simulink model "baselineisp_ref_imp_v1"  (R2023b)
settings: Solver=VariableStepAuto  StartTime=0.0  StopTime=0  RelTol=1e-3
undefined symbols (not defined in the file): gray, ispdata, ispdatainfo
libraries: visionconversions x1, visionanalysis x1
settings Model: Creator=csl  LastModifiedBy=csl

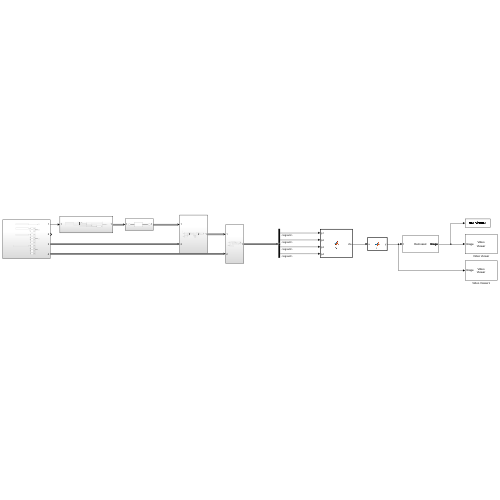
[thumbnail: Simulink's stored preview of the top-level diagram]
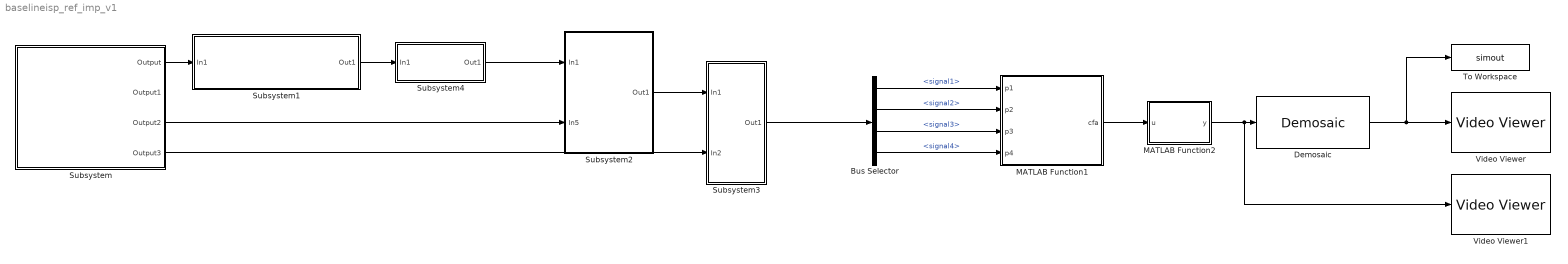
== system baselineisp_ref_imp_v1 ==
  Bus Selector : BusSelector  OutputSignals=signal1,signal2,signal3,signal4
  Demosaic : visionconversions/Demosaic  algorithm=Obsolete  algorithmActive=Bilinear  alignment=BGGR  imagePorts=One multidimensional signal  roundingMode=Floor  overflowMode=on  prodOutputMode=Binary point scaling  prodOutputWordLength=32  prodOutputFracLength=10
  MATLAB Function1 : MATLAB Function  TreatAsAtomicUnit=on
  MATLAB Function2 : MATLAB Function  TreatAsAtomicUnit=on
  Subsystem : Subsystem
  Subsystem1 : Subsystem
  Subsystem2 : Subsystem
  Subsystem3 : Subsystem
  Subsystem4 : Subsystem
  To Workspace : ToWorkspace  VariableName=simout  SaveFormat=Timeseries
  Video Viewer : VideoViewer  colormapValue=gray(256)  FigPos=[1 1078 1093 766]
  Video Viewer1 : VideoViewer  colormapValue=gray(256)  FigPos=[1 1078 1093 766]
  wires:
  Subsystem/3(Output2) -> Subsystem2/2(In5)
  Subsystem2/1(Out1) -> Subsystem3/1(In1)
  Subsystem/4(Output3) -> Subsystem3/2(In2)
  Subsystem3/1(Out1) -> Bus Selector/1
  Bus Selector/1 -> MATLAB Function1/1(p1)  "<signal1>"
  Bus Selector/2 -> MATLAB Function1/2(p2)  "<signal2>"
  Bus Selector/3 -> MATLAB Function1/3(p3)  "<signal3>"
  Bus Selector/4 -> MATLAB Function1/4(p4)  "<signal4>"
  MATLAB Function2/1(y) -> Video Viewer1/1, Demosaic/1
  MATLAB Function1/1(cfa) -> MATLAB Function2/1(u)
  Demosaic/1 -> Video Viewer/1, To Workspace/1
  Subsystem1/1(Out1) -> Subsystem4/1(In1)
  Subsystem/1(Output) -> Subsystem1/1(In1)
  Subsystem4/1(Out1) -> Subsystem2/1(In1)

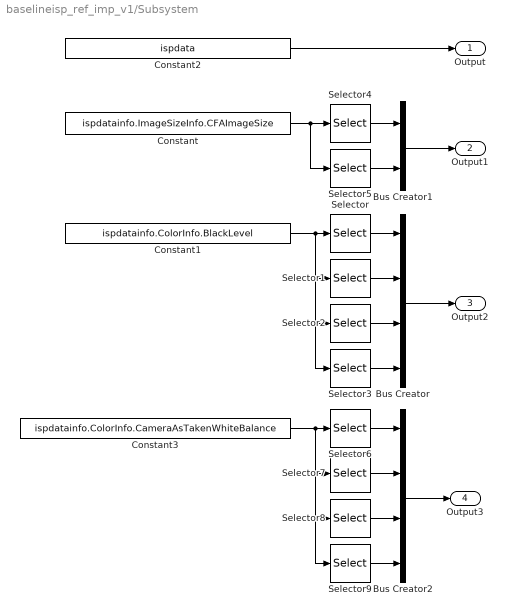
== system baselineisp_ref_imp_v1/Subsystem ==
  Bus Creator : BusCreator  Inputs=4
  Bus Creator1 : BusCreator  Inputs=2
  Bus Creator2 : BusCreator  Inputs=4
  Constant : Constant  Value=ispdatainfo.ImageSizeInfo.CFAImageSize
  Constant1 : Constant  Value=ispdatainfo.ColorInfo.BlackLevel  OutDataTypeStr=uint16
  Constant2 : Constant  Value=ispdata  OutDataTypeStr=uint16
  Constant3 : Constant  Value=ispdatainfo.ColorInfo.CameraAsTakenWhiteBalance  OutDataTypeStr=double
  Selector : Selector  NumberOfDimensions=2  InputPortWidth=3  IndexOptions=Index vector (dialog),Index vector (dialog)  Indices=1,1  OutputSizes=1,1
  Selector1 : Selector  NumberOfDimensions=2  InputPortWidth=3  IndexOptions=Index vector (dialog),Index vector (dialog)  Indices=1,2  OutputSizes=1,1
  Selector2 : Selector  NumberOfDimensions=2  InputPortWidth=3  IndexOptions=Index vector (dialog),Index vector (dialog)  Indices=2,1  OutputSizes=1,1
  Selector3 : Selector  NumberOfDimensions=2  InputPortWidth=3  IndexOptions=Index vector (dialog),Index vector (dialog)  Indices=2,2  OutputSizes=1,1
  Selector4 : Selector  InputPortWidth=2  IndexOptions=Index vector (dialog)  Indices=1  OutputSizes=1
  Selector5 : Selector  InputPortWidth=2  IndexOptions=Index vector (dialog)  Indices=2  OutputSizes=1
  Selector6 : Selector  InputPortWidth=4  IndexOptions=Index vector (dialog)  Indices=1  OutputSizes=1
  Selector7 : Selector  InputPortWidth=4  IndexOptions=Index vector (dialog)  Indices=2  OutputSizes=1
  Selector8 : Selector  InputPortWidth=4  IndexOptions=Index vector (dialog)  Indices=3  OutputSizes=1
  Selector9 : Selector  InputPortWidth=4  IndexOptions=Index vector (dialog)  Indices=4  OutputSizes=1
  Output : Outport
  Output1 : Outport  Port=2
  Output2 : Outport  Port=3
  Output3 : Outport  Port=4
  wires:
  Selector/1 -> Bus Creator/1
  Selector1/1 -> Bus Creator/2
  Selector2/1 -> Bus Creator/3
  Selector3/1 -> Bus Creator/4
  Constant1/1 -> Selector3/1, Selector2/1, Selector1/1, Selector/1
  Selector4/1 -> Bus Creator1/1
  Selector5/1 -> Bus Creator1/2
  Constant/1 -> Selector5/1, Selector4/1
  Bus Creator1/1 -> Output1/1
  Bus Creator/1 -> Output2/1
  Constant2/1 -> Output/1
  Selector6/1 -> Bus Creator2/1
  Selector7/1 -> Bus Creator2/2
  Selector8/1 -> Bus Creator2/3
  Selector9/1 -> Bus Creator2/4
  Constant3/1 -> Selector9/1, Selector8/1, Selector7/1, Selector6/1
  Bus Creator2/1 -> Output3/1

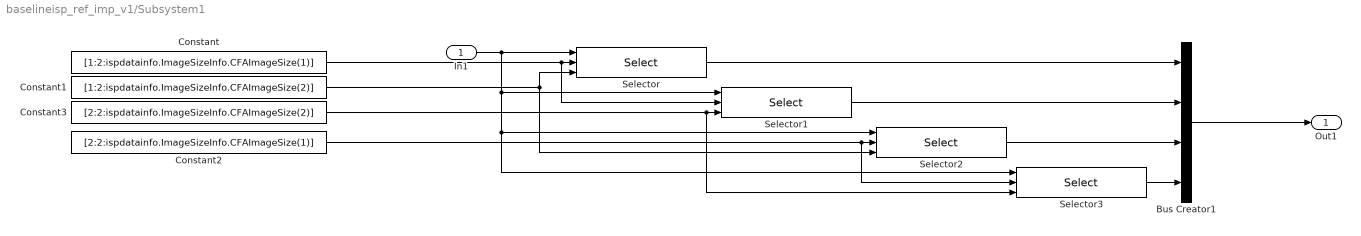
== system baselineisp_ref_imp_v1/Subsystem1 ==
  In1 : Inport
  Bus Creator1 : BusCreator  Inputs=4
  Constant : Constant  Value=[1:2:ispdatainfo.ImageSizeInfo.CFAImageSize(1)]
  Constant1 : Constant  Value=[1:2:ispdatainfo.ImageSizeInfo.CFAImageSize(2)]
  Constant2 : Constant  Value=[2:2:ispdatainfo.ImageSizeInfo.CFAImageSize(1)]
  Constant3 : Constant  Value=[2:2:ispdatainfo.ImageSizeInfo.CFAImageSize(2)]
  Selector{,1..3} (4 alike) : Selector  NumberOfDimensions=2  InputPortWidth=3  IndexOptions=Index vector (port),Index vector (port)  Indices=[1 3],1  OutputSizes=1,1
  Out1 : Outport
  wires:
  Selector1/1 -> Bus Creator1/2
  Selector2/1 -> Bus Creator1/3
  Bus Creator1/1 -> Out1/1
  Selector/1 -> Bus Creator1/1
  Selector3/1 -> Bus Creator1/4
  In1/1 -> Selector/1, Selector2/1, Selector3/1, Selector1/1
  Constant/1 -> Selector1/2, Selector/2
  Constant1/1 -> Selector/3, Selector2/3
  Constant3/1 -> Selector3/3, Selector1/3
  Constant2/1 -> Selector3/2, Selector2/2

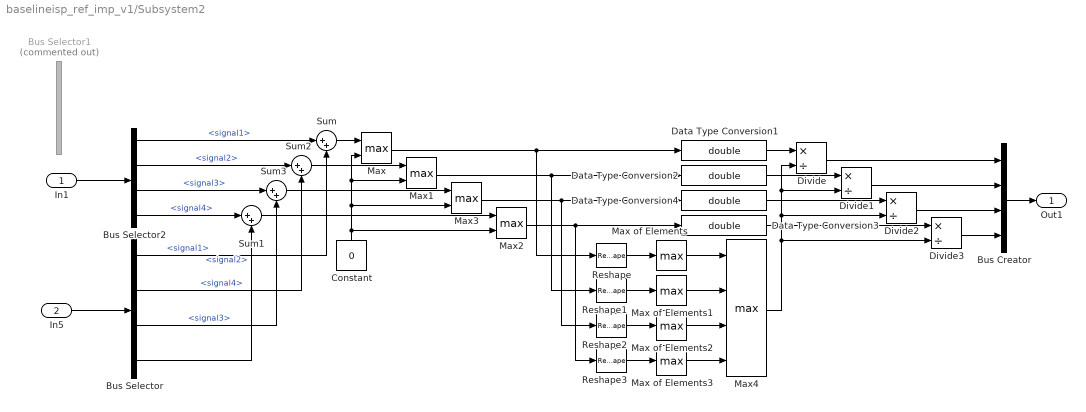
== system baselineisp_ref_imp_v1/Subsystem2 ==
  In1 : Inport
  In5 : Inport  Port=2
  Bus Creator : BusCreator  Inputs=4
  Bus Selector : BusSelector  OutputSignals=signal1,signal4,signal3,signal2
  Bus Selector1 : BusSelector  Commented=on  OutputSignals=p1,p2,p3,p4
  Bus Selector2 : BusSelector  OutputSignals=signal1,signal2,signal3,signal4
  Constant : Constant  Value=0
  Data Type Conversion{1..4} (4 alike) : DataTypeConversion  OutDataTypeStr=double  SaturateOnIntegerOverflow=off  RndMeth=Floor
  Divide{,1..3} (4 alike) : Product  Inputs=*/
  Max{,1..3} (4 alike) : MinMax  Function=max  Inputs=2
  Max of Elements{,1..3} (4 alike) : MinMax  Function=max
  Max4 : MinMax  Function=max  Inputs=4
  Reshape{,1..3} (4 alike) : Reshape
  Sum{,1..3} (4 alike) : Sum  Inputs=|++
  Out1 : Outport
  wires:
  Bus Selector/3 -> Sum3/2  "<signal3>"
  In5/1 -> Bus Selector/1
  Bus Selector/1 -> Sum/2  "<signal1>"
  Bus Selector2/2 -> Sum2/1  "<signal2>"
  Bus Selector/2 -> Sum2/2  "<signal4>"
  Bus Selector2/3 -> Sum3/1  "<signal3>"
  Bus Selector2/4 -> Sum1/1  "<signal4>"
  Bus Selector/4 -> Sum1/2  "<signal2>"
  Bus Selector2/1 -> Sum/1  "<signal1>"
  Bus Creator/1 -> Out1/1
  In1/1 -> Bus Selector2/1
  Sum/1 -> Max/1
  Sum2/1 -> Max1/1
  Sum3/1 -> Max3/1
  Sum1/1 -> Max2/1
  Max/1 -> Reshape/1, Data Type Conversion1/1
  Max1/1 -> Data Type Conversion2/1, Reshape1/1
  Max3/1 -> Data Type Conversion4/1, Reshape2/1
  Max2/1 -> Data Type Conversion3/1, Reshape3/1
  Constant/1 -> Max3/2, Max1/2, Max/2, Max2/2
  Reshape/1 -> Max of Elements/1
  Reshape1/1 -> Max of Elements1/1
  Reshape2/1 -> Max of Elements2/1
  Reshape3/1 -> Max of Elements3/1
  Max of Elements/1 -> Max4/1
  Max of Elements1/1 -> Max4/2
  Max of Elements2/1 -> Max4/3
  Max of Elements3/1 -> Max4/4
  Data Type Conversion2/1 -> Divide1/1
  Data Type Conversion4/1 -> Divide2/1
  Data Type Conversion1/1 -> Divide/1
  Data Type Conversion3/1 -> Divide3/1
  Divide/1 -> Bus Creator/1
  Divide1/1 -> Bus Creator/2
  Divide2/1 -> Bus Creator/3
  Divide3/1 -> Bus Creator/4
  Max4/1 -> Divide3/2, Divide2/2, Divide1/2, Divide/2

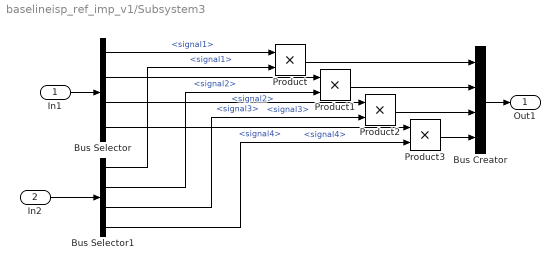
== system baselineisp_ref_imp_v1/Subsystem3 ==
  In1 : Inport
  In2 : Inport  Port=2
  Bus Creator : BusCreator  Inputs=4
  Bus Selector : BusSelector  OutputSignals=signal1,signal2,signal3,signal4
  Bus Selector1 : BusSelector  OutputSignals=signal1,signal2,signal3,signal4
  Product{,1..3} (4 alike) : Product
  Out1 : Outport
  wires:
  Product3/1 -> Bus Creator/4
  Product1/1 -> Bus Creator/2
  Product2/1 -> Bus Creator/3
  Product/1 -> Bus Creator/1
  In2/1 -> Bus Selector1/1
  In1/1 -> Bus Selector/1
  Bus Creator/1 -> Out1/1
  Bus Selector/1 -> Product/1  "<signal1>"
  Bus Selector/2 -> Product1/1  "<signal2>"
  Bus Selector/3 -> Product2/1  "<signal3>"
  Bus Selector/4 -> Product3/1  "<signal4>"
  Bus Selector1/1 -> Product/2  "<signal1>"
  Bus Selector1/2 -> Product1/2  "<signal2>"
  Bus Selector1/3 -> Product2/2  "<signal3>"
  Bus Selector1/4 -> Product3/2  "<signal4>"

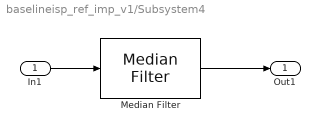
== system baselineisp_ref_imp_v1/Subsystem4 ==
  In1 : Inport
  Median Filter : visionanalysis/Median Filter  nghbood=[3 3]  outSize=Same as input port I  padType=Symmetric  padSrc=Specify via dialog  padVal=0  roundingMode=Floor  overflowMode=off
  Out1 : Outport
  wires:
  In1/1 -> Median Filter/1
  Median Filter/1 -> Out1/1

== matlab function baselineisp_ref_imp_v1/MATLAB Function1 ==
  data: p1 input; cfa output; p2 input; p3 input; p4 input
function cfa = fcn(p1,p2,p3,p4)
    outHeight = 2*size(p1, 1);
    outWidth = 2*size(p1, 2);
    cfa = zeros([outHeight outWidth]);
    cfa(1:2:end, 1:2:end) = p1;
    cfa(1:2:end, 2:2:end) = p2;
    cfa(2:2:end, 1:2:end) = p3;
    cfa(2:2:end, 2:2:end) = p4;
end

== matlab function baselineisp_ref_imp_v1/MATLAB Function2 ==
  data: u input; y output
function y = fcn(u)
y = im2uint16(u);
end
